simulink model "W02_MSD_ThreeWays"  (R2024b)
settings: Solver=ode45  StartTime=0.0  StopTime=t_end  MaxStep=0.01  RelTol=1e-3
PreLoadFcn:
  | % W02_MSD_ThreeWays 기본 파라미터 (모델을 열 때 자동 실행)
  | % 이미 워크스페이스에 값이 있으면 그대로 두고, 없을 때만 채웁니다.
  | defs = { 'm',1 ; 'b',0.2 ; 'k',1 ; 'F_amp',1 ; 't_end',40 ;
  |          'x0_pos',0 ; 'x0_vel',0 ;
  |          'A_msd',[0 1; -1 -0.2] ; 'B_msd',[0;1] ;
  |          'C_msd',[1 0] ; 'D_msd',0 };
  | for ii = 1:size(defs,1)
  |     if ~evalin('base', sprintf('exist(''%s'',''var'')', defs{ii,1}))
  |         assignin('base', defs{ii,1}, defs{ii,2});
  |     end
  | end
  | clear defs ii
values from neighbouring files (symbols this model uses):
  A_msd = p.A    [W02_03_run_simulink.m]
  b = 0.2    [W02_02_msd_derivation.m]    (also in W02_03_run_simulink.m = p.b; W02_04_ss_tf_conversion.m = p.b)
  B_msd = p.B    [W02_03_run_simulink.m]
  C_msd = p.C    [W02_03_run_simulink.m]
  D_msd = p.D    [W02_03_run_simulink.m]
  F_amp = 0    [W02_03_run_simulink.m]
  k = 1.0    (= 1)    [W02_02_msd_derivation.m]    (also in W02_03_run_simulink.m = p.k; W02_04_ss_tf_conversion.m = p.k)
  m = 1.0    (= 1)    [W02_02_msd_derivation.m]    (also in W02_03_run_simulink.m = p.m; W02_04_ss_tf_conversion.m = p.m)
  x0_pos = 0.5    [W02_03_run_simulink.m]
  x0_vel = 0    [W02_03_run_simulink.m]
settings Model: Creator=admin  LastModifiedBy=admin

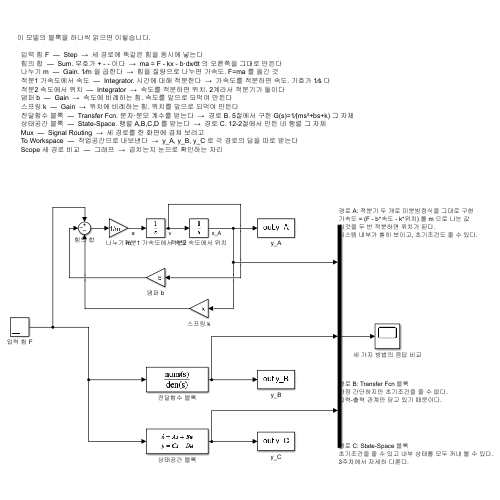
[thumbnail: Simulink's stored preview of the top-level diagram]
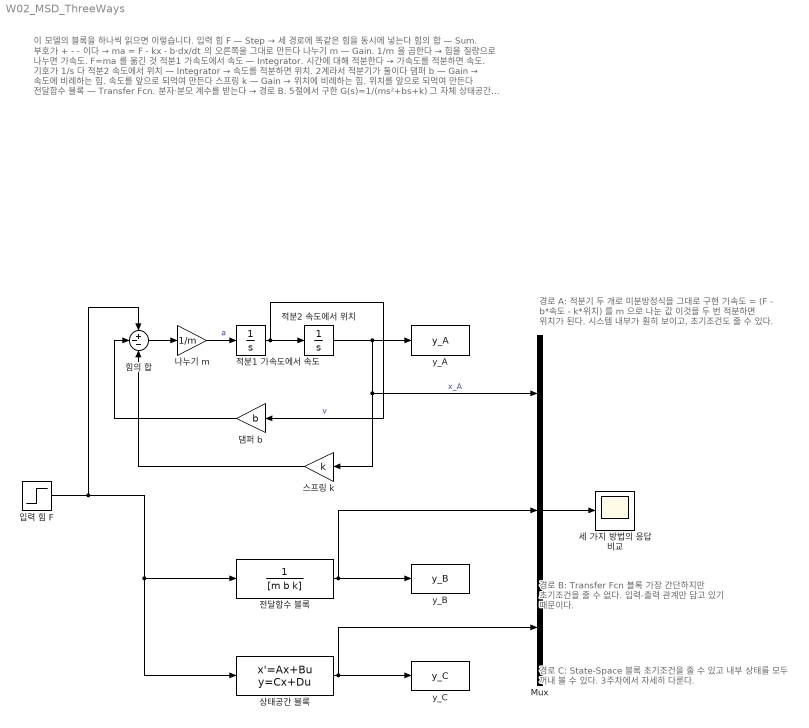
== system W02_MSD_ThreeWays ==
  note: 경로 A: 적분기 두 개로 미분방정식을 그대로 구현
      | 가속도 = (F - b*속도 - k*위치) 를 m 으로 나눈 값
      | 이것을 두 번 적분하면 위치가 된다.
      | 시스템 내부가 훤히 보이고, 초기조건도 줄 수 있다.
  note: 경로 B: Transfer Fcn 블록
      | 가장 간단하지만 초기조건을 줄 수 없다.
      | 입력-출력 관계만 담고 있기 때문이다.
  note: 경로 C: State-Space 블록
      | 초기조건을 줄 수 있고 내부 상태를 모두 꺼내 볼 수 있다.
      | 3주차에서 자세히 다룬다.
  note: 이 모델의 블록을 하나씩 읽으면 이렇습니다.
      |
      |   입력 힘 F  —  Step  →  세 경로에 똑같은 힘을 동시에 넣는다
      |   힘의 합  —  Sum. 부호가 + - - 이다  →  ma = F - kx - b·dx∕dt 의 오른쪽을 그대로 만든다
      |   나누기 m  —  Gain. 1∕m 을 곱한다  →  힘을 질량으로 나누면 가속도. F=ma 를 옮긴 것
      |   적분1 가속도에서 속도  —  Integrator. 시간에 대해 적분한다  →  가속도를 적분하면 속도. 기호가 1∕s 다
      |   적분2 속도에서 위치  —  Integrator  →  속도를 적분하면 위치. 2계라서 적분기가 둘이다
      |   댐퍼 b  —  Gain  →  속도에 비례하는 힘. 속도를 앞으로 되먹여 만든다
      |   스프링 k  —  Gain  →  위치에 비례하는 힘. 위치를 앞으로 되먹여 만든다
      |   전달함수 블록  —  Transfer Fcn. 분자·분모 계수를 받는다  →  경로 B. 5절에서 구한 G(s)=1∕(ms²+bs+k) 그 자체
      |   상태공간 블록  —  State-Space. 행렬 A,B,C,D 를 받는다  →  경로 C. 12-2절에서 만든 네 행렬 그 자체
      |   Mux  —  Signal Routing  →  세 경로를 한 화면에 겹쳐 보려고
      |   To Workspace  —  작업공간으로 내보낸다  →  y_A, y_B, y_C 로 각 경로의 답을 따로 받는다
      |   Scope 세 경로 비교  —  그래프  →  겹치는지 눈으로 확인하는 자리
  Mux : Mux  Inputs=3
  y_A : ToWorkspace  VariableName=y_A  SaveFormat=Timeseries  SampleTime=-1
  y_B : ToWorkspace  VariableName=y_B  SaveFormat=Timeseries  SampleTime=-1
  y_C : ToWorkspace  VariableName=y_C  SaveFormat=Timeseries  SampleTime=-1
  나누기 m : Gain  Gain=1/m
  댐퍼 b : Gain  Gain=b
  상태공간 블록 : StateSpace  A=A_msd  B=B_msd  C=C_msd  D=D_msd  InitialCondition=[x0_pos; x0_vel]
  세 가지 방법의 응답 비교 : Scope
  스프링 k : Gain  Gain=k
  입력 힘 F : Step  Time=0  After=F_amp  SampleTime=0
  적분1 가속도에서 속도 : Integrator  InitialCondition=x0_vel
  적분2 속도에서 위치 : Integrator  InitialCondition=x0_pos
  전달함수 블록 : TransferFcn  Denominator=[m b k]
  힘의 합 : Sum  Inputs=+--
  wires:
  입력 힘 F/1 -> 상태공간 블록/1, 전달함수 블록/1, 힘의 합/1
  힘의 합/1 -> 나누기 m/1
  나누기 m/1 -> 적분1 가속도에서 속도/1  "a"
  적분1 가속도에서 속도/1 -> 적분2 속도에서 위치/1, 댐퍼 b/1  "v"
  댐퍼 b/1 -> 힘의 합/2
  적분2 속도에서 위치/1 -> Mux/1, 스프링 k/1, y_A/1  "x_A"
  스프링 k/1 -> 힘의 합/3
  전달함수 블록/1 -> y_B/1, Mux/2
  상태공간 블록/1 -> y_C/1, Mux/3
  Mux/1 -> 세 가지 방법의 응답 비교/1
